simulink model "Simplified_asynchronous1"  (R2022b)
settings: Solver=VariableStepAuto  StartTime=0.0  StopTime=25  RelTol=1e-3
libraries: spsACVoltageSourceLib x3, spsAsynchronousMachineSIUnitsLib x1, spsGroundLib x1, sps_lib x1
settings Model: Creator=Hessam  LastModifiedBy=Hessam

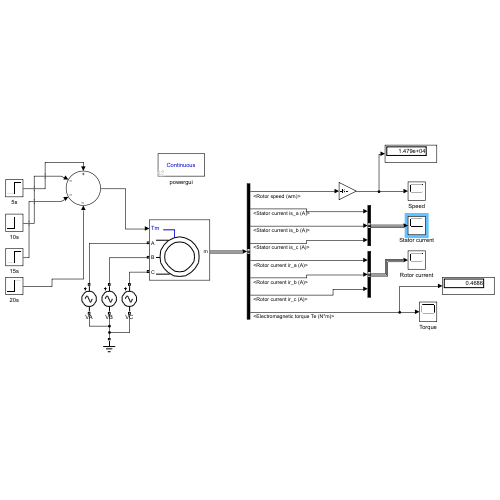
[thumbnail: Simulink's stored preview of the top-level diagram]
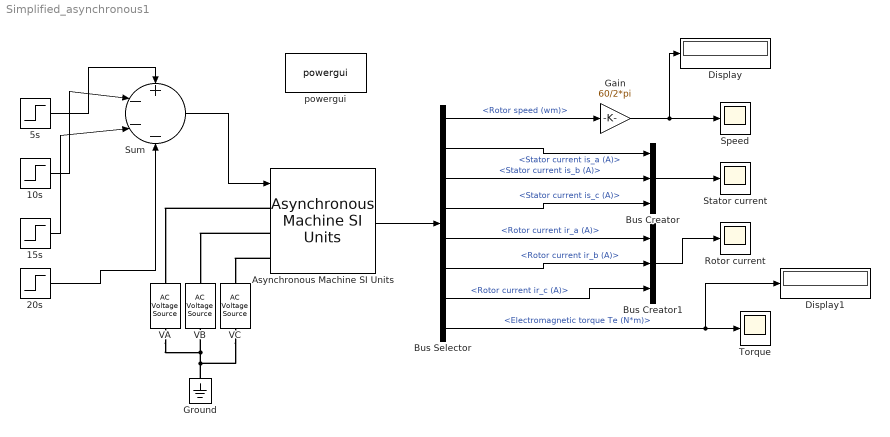
== system Simplified_asynchronous1 ==
  10s : Step  Time=10  After=13.36  SampleTime=0
  15s : Step  Time=15  After=6.68  SampleTime=0
  20s : Step  Time=20  After=6.68  SampleTime=0
  5s : Step  Time=5  After=26.72  SampleTime=0
  Asynchronous Machine SI Units : spsAsynchronousMachineSIUnitsLib/Asynchronous Machine SI Units  RotorType=Squirrel-cage  PresetModel="15:  5.4 HP (4KW)   400 V  50Hz 1430 RPM"  MechanicalLoad=Torque Tm  ShowDetailedParameters=on  ReferenceFrame=Rotor  Units=SI  MeasurementBus=off  NominalParameters=[4000 400 50]  VoltageRatio=1  Stator=[1.405 0.005839]  Rotor=[1.395 0.005839]  Cage1=[0.4155 0.002066]  Cage2=[0.4168 0.0003495]  Lm=0.1722  Mechanical=[0.0131 0.002985 2]  PolePairs=2  InitialConditions=[0 0 0 0 0 0 0 0]  SimulateSaturation=off  Saturation=[14.03593122, 27.81365428, 53.79336849, 72.68890987, 97.98006896, 148.6815601, 215.7428561, 302.9841135, 428.7778367 ; 230, 322, 414, 460, 506, 552, 598, 644, 690]  LoadFlowParameters=1492000  TsPowergui=0  TsBlock=-1  IterativeModel=Trapezoidal non iterative  IterativeDiscreteModel=Trapezoidal non iterative  Pmec=1.492e+006
  Bus Creator : BusCreator  Inputs=3
  Bus Creator1 : BusCreator  Inputs=3
  Bus Selector : BusSelector  OutputSignals=Mechanical.Rotor speed (wm),Stator measurements.Stator current is_a (A),Stator measurements.Stator current is_b (A),Stator measurements.Stator current is_c (A),Rotor measurements.Rotor current ir_a (A),Rotor measurements.Rotor current ir_b (A),Rotor measurements.Rotor current ir_c (A),Mechanical.Electromagnetic torque Te (N*m)
  Display : Display
  Display1 : Display
  Gain : Gain  Gain=60/2*pi
  Ground : spsGroundLib/Ground  LConnTagsString=a
  Rotor current : Scope
  Speed : Scope
  Stator current : Scope
  Sum : Sum  Inputs=+---
  Torque : Scope
  VA : spsACVoltageSourceLib/AC Voltage Source  Amplitude=326.59  Phase=0  Frequency=50  SampleTime=0  Measurements=None  BusType=swing  Pref=10e3  Qref=0  Qmin=-inf  Qmax=+inf
  VB : spsACVoltageSourceLib/AC Voltage Source  Amplitude=326.59  Phase=-120  Frequency=50  SampleTime=0  Measurements=None  BusType=swing  Pref=10e3  Qref=0  Qmin=-inf  Qmax=+inf
  VC : spsACVoltageSourceLib/AC Voltage Source  Amplitude=326.59  Phase=120  Frequency=50  SampleTime=0  Measurements=None  BusType=swing  Pref=10e3  Qref=0  Qmin=-inf  Qmax=+inf
  powergui : sps_lib/powergui  Priority=1  SimulationMode=Continuous  SampleTime=50e-6  frequency=60  Iterations=50  frequencyindice=50  Pbase=100e6  ErrMax=1e-4  UnitsV=kV  UnitsW=MW  buscounter=0  FunctionMessages=off  echomessages=off  EnableUseOfTLC=off  CurrentSourceSwitches=off  DisableSnubberDevices=off  DisableRonSwitches=off  DisableVfSwitches=off  DisplayEquations=off  AutomaticDiscreteSolvers=off  SolverType=Tustin/Backward Euler (TBE)  Interpol=off  ExternalGateDelay=off  methode=off  Ts=100  x0status=blocks  SPID=on  SwTol=0  HookPort=off  NonlinearTolerance=1e-4  nMaxIteration=100  ContinueOnMaxIteration=off  RestoreLinks=warning  ResistiveCurrentMeasurement=off  Frange=[0:2:500]  Ylog=off  Xlog=on  ShowGrid=off  save=off  variable=ZData  structure=0  ZoomFFT=off  StartTime=0.0  cycles=1  DisplayStyle=1  fundamental=60  FreqAxis=off  MaxFrequency=1000  frequencyindicesteady=1  RmsSteady=1  display=off
  wires:
  Asynchronous Machine SI Units/1 -> Bus Selector/1
  Bus Selector/1 -> Gain/1  "<Rotor speed (wm)>"
  Gain/1 -> Display/1, Speed/1
  Bus Selector/8 -> Torque/1, Display1/1  "<Electromagnetic torque Te (N*m)>"
  Bus Selector/2 -> Bus Creator/1  "<Stator current is_a (A)>"
  Bus Selector/3 -> Bus Creator/2  "<Stator current is_b (A)>"
  Bus Selector/4 -> Bus Creator/3  "<Stator current is_c (A)>"
  Bus Selector/5 -> Bus Creator1/1  "<Rotor current ir_a (A)>"
  Bus Selector/6 -> Bus Creator1/2  "<Rotor current ir_b (A)>"
  Bus Selector/7 -> Bus Creator1/3  "<Rotor current ir_c (A)>"
  Bus Creator/1 -> Stator current/1
  Bus Creator1/1 -> Rotor current/1
  5s/1 -> Sum/1
  Sum/1 -> Asynchronous Machine SI Units/1
  10s/1 -> Sum/2
  15s/1 -> Sum/3
  20s/1 -> Sum/4
  connections:
  Asynchronous Machine SI Units/LConn1 -- VA/RConn1
  Asynchronous Machine SI Units/LConn2 -- VB/RConn1
  Asynchronous Machine SI Units/LConn3 -- VC/RConn1
  Ground/LConn1 -- VC/LConn1 -- VA/LConn1 -- VB/LConn1
